simulink model "item2"  (R2013a)
settings: Solver=ode45  StartTime=0.0  StopTime=1  RelTol=1e-3
libraries: powerlib x4
settings Model: Creator=Guilherme  LastModifiedBy=Guilherme

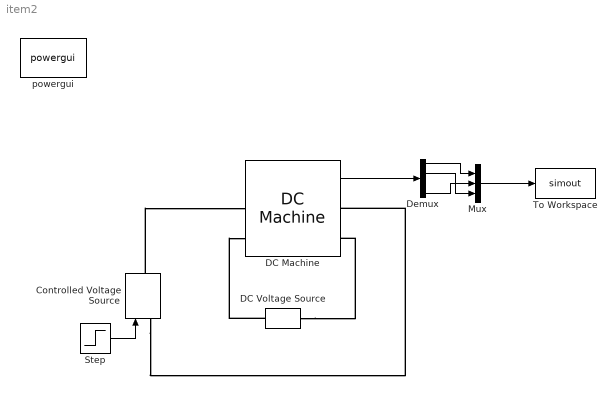
== system item2 ==
  Controlled Voltage Source : powerlib/Electrical Sources/Controlled Voltage Source  Initialize=on  Source_Type=AC  Amplitude=0  Phase=0  Frequency=0  Measurements=None
  DC Machine : powerlib/Machines/DC Machine  PresetModel=No  MechanicalLoad=Torque TL  FieldType=Wound  ShowDetailedParameters=on  RLa="[ 1.6  6.67e-4 ]"  RLf=[ 1 0 ]  Laf=0.038  MachineConstant=Torque constant (N.m/A)  Ke=1.8  Kt=1.8  J=1.1e-4  Bm=1.24e-4  Tf=0  w0=1  Ifinit=1  TsPowergui=0  TsBlock=-1
  DC Voltage Source : powerlib/Electrical Sources/DC Voltage Source  Amplitude=1  Measurements=None
  Demux : Demux
  Mux : Mux  Inputs=3
  Step : Step  Time=0.1  After=24  SampleTime=0
  To Workspace : ToWorkspace  VariableName=simout  SampleTime=-1  SaveFormat=Timeseries
  powergui : powerlib/powergui  Priority=1  SimulationMode=Discrete  SolverType=Tustin  SampleTime=50e-6  frequency=60  SPID=off  DisableSnubberDevices=off  DisableRonSwitches=off  DisableVfSwitches=off  SwTol=0  Interpol=off  DisplayEquations=off  frequencyindice=0  Pbase=100e6  ErrMax=1e-4  Iterations=50  UnitsV=kV  UnitsW=MW  FunctionMessages=off  echomessages=off  HookPort=off  EnableUseOfTLC=off  x0status=blocks  RestoreLinks=warning  ResistiveCurrentMeasurement=off  Frange=[0:2:500]  Ylog=off  Xlog=on  ShowGrid=off  save=off  variable=ZData  ZoomFFT=off  StartTime=0.0  cycles=1  DisplayStyle=1  fundamental=60  FreqAxis=off  MaxFrequency=1000  frequencyindicesteady=1  RmsSteady=1  display=off  Ts=0  methode=off
  wires:
  Step/1 -> Controlled Voltage Source/1
  DC Machine/1 -> Demux/1
  Mux/1 -> To Workspace/1
  Demux/1 -> Mux/1
  Demux/2 -> Mux/3
  Demux/4 -> Mux/2
  connections:
  DC Voltage Source/RConn1 -- DC Machine/LConn2
  DC Voltage Source/LConn1 -- DC Machine/RConn2
  Controlled Voltage Source/RConn1 -- DC Machine/LConn1
  Controlled Voltage Source/LConn1 -- DC Machine/RConn1
